simulink model "elevation_model"  (R2021b)
settings: Solver=VariableStepAuto  StartTime=0.0  StopTime=45  RelTol=1e-3
values from neighbouring files (symbols this model uses):
  ts3 = 10^-3    (= 0.001)    [loading_project.m]
libraries: simulink x3
settings Model: Creator=noait  LastModifiedBy=noait

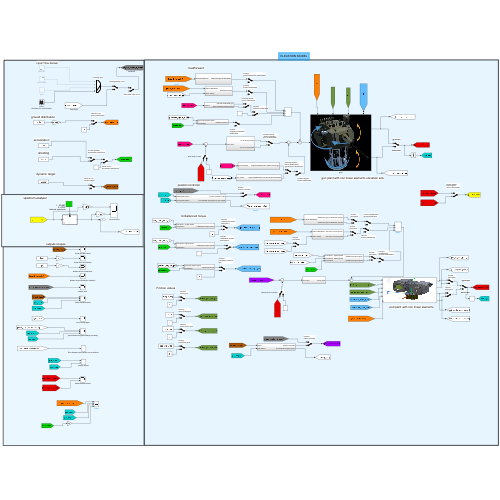
[thumbnail: Simulink's stored preview of the top-level diagram]
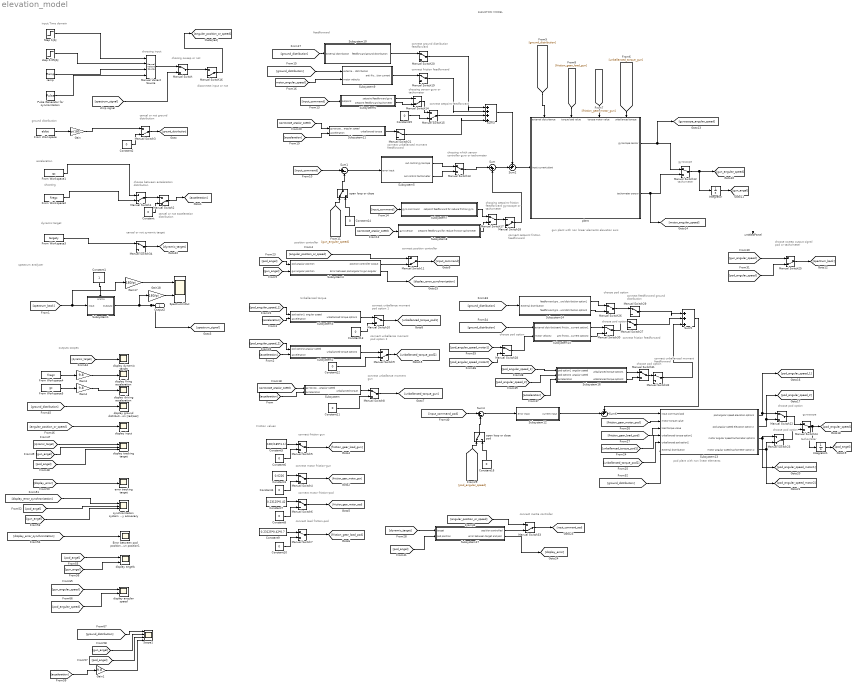
== system elevation_model ==
  note: ELEVATION MODEL
  note: outputs scopes
  note: connect
      | friction feedforward
  note: connect feedforward
      | ground distribution
  note: choose
      | pod option
  note: connect
      | unballance moment
      | pod option 2
  note: connect
      | inertia controller
  note: connect
      | motor friction-gun
  note: connect
      | friction gun
  note: choose sweep
      | output signal
      |  pod or tachometer
  note: connect
      | position controller
  note: connect setpoint
      | friction feedforward
  note: chossing setpoint
      | friction feedforward
      |  gyroscope or tachometer
  note: chossing which
      |  sensor controller
      | gyro or tachometer
  note: chossing sensor
      | gyro or tachometer
  note: connect
      | ground distribution feedforward
  note: disconnect input or not
  note: chosing sweep or not
  note: choosing input
  note: cancel or not
      | synamic target
  note: cancel or not
      | ground distribution
  note: cancel or not
      | acceleration distribution
  note: choose between
      | acceleration distribution
  note: pod plant with non linear elements
  note: dynamic target
  note: feedforward
  note: shooting
  note: position controller
  note: gun plant with non linear elements elevation axis
  note: tachometer
  note: gyroscope
  note: Unballanced torque
  note: Friction values
  note: acceleration
  note: ground distribution
  note: spectrum analyzer
  note: input:Time domain
  note: connect
      | friction feedforward
  note: connect
      | setpoint feedforward
  note: connect
      | unballanced moment
      | feedforward
  note: connect
      | motor friction-pod
  note: connect
      | load friction-pod
  note: connect
      | unballance moment
      | pod option 1
  note: connect
      | unballance moment
      | gun
  note: choose
      | pod option
  note: choose
      | pod option
  note: choose
      | pod option
  note: connect
      | unballanced
      | moment feedforward
  note: choose
      | pod option
  note: choose
      | pod option
  note: gyroscope
  note: tachometer
  " synchronization system stability accuaracy" : Scope  NumInputPorts=3
  Constant : Constant  Value=0  SampleTime=-1
  Constant1 : Constant  OutDataTypeStr=boolean
      settings: AttributesFormatString=1 - START\n0 -STOP\ninternal spectrum
      settings: OpenFcn=|
      | if get_param(gcbh,'value')-48 set_param(gcbh,'value','0','backgroundcolor','red');
      | else set_param(gcbh,'value','1','backgroundcolor','green');
      | end
  Constant{4,6,8,10..16} (10 alike) : Constant  Value=0  SampleTime=0
  Constant2 : Constant  Value=0  SampleTime=-1
  Constant3 : Constant  Value=0.0226  SampleTime=0
  Constant5 : Constant  Value=100/(185*1.1)  SampleTime=0
  Constant7 : Constant  Value=0.23125*0.42  SampleTime=0
  Constant9 : Constant  Value=0.23125*0.42*0.7  SampleTime=0
  Error between pod position to gun position1 : Scope
  From Workspace : FromWorkspace  VariableName=eldist  SampleTime=ts3/3  Interpolate=off  ZeroCross=off  OutputAfterFinalValue=Setting to zero
  From Workspace1 : FromWorkspace  VariableName=gz  SampleTime=ts3/3  Interpolate=off  ZeroCross=off  OutputAfterFinalValue=Setting to zero
  From Workspace2 : FromWorkspace  VariableName=firegz  SampleTime=ts3/9  Interpolate=off  ZeroCross=off  OutputAfterFinalValue=Setting to zero
  From Workspace3 : FromWorkspace  VariableName=targety  SampleTime=5*ts3  Interpolate=off  ZeroCross=off  OutputAfterFinalValue=Setting to zero
  From Workspace4 : FromWorkspace  VariableName=firegz  SampleTime=ts3/9  Interpolate=off  ZeroCross=off  OutputAfterFinalValue=Setting to zero
  From Workspace5 : FromWorkspace  VariableName=gz  SampleTime=ts3/3  Interpolate=off  ZeroCross=off  OutputAfterFinalValue=Setting to zero
  Gain : Gain  Gain=pi/180
  Gain1 : Gain  Gain=9.8
  Gain17 : Gain  Gain=180/pi
  Gain18 : Gain  Gain=180/pi
  Gain3 : Gain  Gain=9.8
  Gain4 : Gain  Gain=9.8
  Integrator : Integrator  ZeroCross=off
  Integrator1 : Integrator  ZeroCross=off
  Manual Variant Source : simulink/Signal Routing/Manual Variant Source  NumChoices=4  LabelModeActiveChoice=V_4
  Manual Switch{,4..8,10,12..13,17,19..22,24,26..32,34} (23 alike) : ManualSwitch
  Manual Switch{1..3,9,11,14..16,18,23,25,33} (12 alike) : ManualSwitch  CurrentSetting=0
  Pulse Generator for syncronization : DiscretePulseGenerator  PulseType=Time based  Period=5  PulseWidth=20
  Scope1 : Scope  NumInputPorts=4
  SpectrumInOut : Scope  NumInputPorts=2
  Step 1[A] : Step  SampleTime=0  ZeroCross=off
  Subsystem : Subsystem
  Subsystem1 : Subsystem  mask{GAIN=0.05%2*pi/180%0.5*pi/180, InitFreq=1, TargetTime=500, FreqAtTime=500}
      mask prompts: InitFreq "INITIAL FREQUENCY"; TargetTime "Target Time"; FreqAtTime "Frequency at Time"
  Subsystem10 : Subsystem
  Subsystem11 : Subsystem
  Subsystem12 : Subsystem
  Subsystem13 : Subsystem
      mask Display: image('C:\Users\noait\OneDrive\Desktop\צילום מסך 2024-04-08 195106.png'); % Use "Edit Image" on toolstrip to change.
  Subsystem14 : Subsystem
  Subsystem15 : Subsystem
  Subsystem16 : Subsystem
  Subsystem17 : Subsystem
  Subsystem2 : Subsystem
  Subsystem3 : Subsystem
  Subsystem4 : Subsystem
  Subsystem5 : Subsystem
  Subsystem6 : Subsystem
  Subsystem7 : Subsystem
  Subsystem8 : Subsystem
  Subsystem9 : Subsystem
  Sum : Sum  Inputs=|++
  Sum1 : Sum  Inputs=|+-
  Sum2 : Sum  Inputs=++|
  Sum3 : Sum  Inputs=|++++
  Sum4 : Sum  Inputs=|+-
  Sum5 : Sum  Inputs=|+++
  Sum6 : Sum  Inputs=++|
  display angels : Scope  NumInputPorts=2
  display angular speed : Scope  NumInputPorts=2
  display driving acceleration : Scope
  display dynamic target : Scope
  display firing acceleration : Scope
  display ground distribution [rad/sec] : Scope
  display input : Scope
  display tracking target : Scope  NumInputPorts=3
  error tracking target : Scope
  open loop or close : ManualSwitch
  open loop or close pod : ManualSwitch
  plant : Subsystem  Description=elevation-plant
      settings: PortSchema="{\"entries\":[{\"content\":{\"sides\":[{\"content\":{\"connectorIds\":[\"In1\"]},\"type\":\"ConnectorPlacement.EquallySpacedRectSide\",\"uuid\":\"e984d65b-c4b2-4f64-9138-3f858c9b51b0\"},{\"content\":{\"connectorIds\":[\"Out1\",\"Out2\"],\"side\":\"RIGHT\"},\"type\":\"ConnectorPlacement.EquallySpacedRectSide\",\"uuid\":\"67e0a38d-5f11-4d68-ba2b-c2f31a8ec962\"},{\"content\":{\"connectorIds\":[\"In2\",\"In3\",\"In4\",\"In5\"],\"side\":\"TOP\"},\"type\":\"ConnectorPlacement.EquallySpacedRectSide\",\"uuid\":\"636aa855-affb-4e96-b788-9501fa5a8af5\"}]},\"type\":\"ConnectorPlacement.EquallySpacedConnector\",\"uuid\":\"459d9826-6541-4e32-b3aa-984fb23680a1\"}],\"packageUris\":[\"http://schema.mathworks.com/mf0/Connector/R2020b\"],\"version\":\"1.0\"}"
      mask Display: image('C:\Users\noait\OneDrive\Desktop\צילום.png'); % Use "Edit Image" on toolstrip to change.
  ramp : simulink/Sources/Ramp  slope=1  start=0  InitialOutput=0
  step 0.05[A] : Step  After=0.05  SampleTime=0  ZeroCross=off
  untitledPanel : Subsystem  Tag=HiddenForWebPanel  IsWebBlockPanel=on
  Output2 : Outport
  wires:
  ramp/1 -> Manual Variant Source/3
  Step 1[A]/1 -> Manual Variant Source/1
  Pulse Generator for syncronization/1 -> Manual Variant Source/4
  step 0.05[A]/1 -> Manual Variant Source/2
  Manual Variant Source/1 -> Manual Switch/1
  Gain17/1 -> SpectrumInOut/1
  Constant1/1 -> Subsystem1/Enable
  Subsystem1/1(Output2) -> [spectrum_signal], Output2/1, Gain18/1
  [spectrum_back] -> Gain17/1, Subsystem1/1(Input)
  Gain18/1 -> SpectrumInOut/2
  [spectrum_signal] -> Manual Switch/2
  From Workspace/1 -> Gain/1
  Gain/1 -> Manual Switch3/1
  From Workspace1/1 -> Manual Switch1/1
  From Workspace2/1 -> Manual Switch1/2
  Manual Switch1/1 -> Manual Switch2/1
  Manual Switch2/1 -> [acceleration]
  Constant/1 -> Manual Switch2/2
  Manual Switch3/1 -> [ground_distribution]
  Constant2/1 -> Manual Switch3/2
  Constant3/1 -> Manual Switch4/1
  Constant4/1 -> Manual Switch4/2
  Manual Switch4/1 -> [friction_gear_motor_gun]
  Constant5/1 -> Manual Switch5/1
  Manual Switch5/1 -> [friction_gear_load_gun]
  Constant6/1 -> Manual Switch5/2
  Constant7/1 -> Manual Switch6/1
  Manual Switch6/1 -> [friction_gear_motor_pod]
  Constant8/1 -> Manual Switch6/2
  Manual Switch7/1 -> [friction_gear_load_pod]
  Constant10/1 -> Manual Switch7/2
  Constant9/1 -> Manual Switch7/1
  [acceleration] -> Subsystem/2(acceleration)
  Manual Switch8/1 -> [unballanced_torque_gun]
  Subsystem/1(unballanced torque) -> Manual Switch8/1
  Constant11/1 -> Manual Switch8/2
  Constant12/1 -> Manual Switch9/2
  [acceleration] -> Subsystem2/2(acceleration)
  Subsystem2/1(unballanced torque option2) -> Manual Switch9/1
  Constant13/1 -> Manual Switch10/2
  [acceleration] -> Subsystem3/2(acceleration)
  Subsystem3/1(unballanced torque option1) -> Manual Switch10/1
  Manual Switch10/1 -> [unballanced_torque_pod1]
  Manual Switch9/1 -> [unballanced_torque_pod2]
  Subsystem4/1(position controller output) -> Manual Switch11/2
  [angular_position_or_speed] -> Manual Switch11/1
  Manual Switch11/1 -> [input_command]
  [unballanced_torque_gun] -> plant/5(unballanced torque)
  [friction_gear_motor_gun] -> plant/4(torque motor value)
  [friction_gear_load_gun] -> plant/3(torque load value)
  plant/2(tachometer sensor) -> [motor_angular_speed], Manual Switch12/2
  plant/1(gyroscope sensor) -> [gyroscope_angular_speed], Manual Switch12/1
  Manual Switch12/1 -> Integrator/1, [gun_angular_speed]
  Integrator/1 -> [gun_angel]
  [gun_angel] -> Subsystem4/2(gun angular position)
  Subsystem5/1(out control gyroscope) -> Manual Switch13/1
  Subsystem5/2(out control tachometer) -> Manual Switch13/2
  Sum1/1 -> Subsystem5/1(error input)
  [input_command] -> Sum1/1
  open loop or close/1 -> Sum1/2
  [gun_angular_speed] -> open loop or close/1
  Constant14/1 -> open loop or close/2
  Subsystem6/1(setpoind feedforward gyro) -> Manual Switch14/1
  Subsystem6/2(setpoint feedforward tachometer) -> Manual Switch14/2
  Manual Switch14/1 -> Manual Switch15/1
  Constant15/1 -> Manual Switch15/2
  Manual Switch/1 -> Manual Switch16/1
  Manual Switch16/1 -> [angular_position_or_speed]
  Sum/1 -> Sum2/2
  Sum2/1 -> plant/1(input current plant)
  [gyroscope_angular_speed] -> Subsystem8/1(gyro sensor)
  Subsystem8/1(setpoint feedforward for reduce friction tachometer) -> Manual Switch17/2
  Subsystem7/1(setpoint feedforward for reduce friction gyro) -> Manual Switch17/1
  Manual Switch17/1 -> Manual Switch18/1
  Manual Switch13/1 -> Sum/1
  Manual Switch18/1 -> Sum/2
  [input_command] -> Subsystem6/1(setpoint)
  [input_command] -> Subsystem7/1(gyro command)
  [ground_distribution] -> Subsystem9/1(external distribution)
  Subsystem9/1(anti friction current) -> Manual Switch19/1
  Sum3/1 -> Sum2/1
  [motor_angular_speed] -> Subsystem9/2(motor velocity)
  [ground_distribution] -> Subsystem10/1(external distribution)
  Subsystem10/1(feedforward ground distribution) -> Manual Switch20/1
  Manual Switch20/1 -> Sum3/1
  Manual Switch19/1 -> Sum3/2
  Manual Switch15/1 -> Sum3/3
  [gyroscope_angular_speed] -> Subsystem/1(gyroscope angular speed)
  [gyroscope_angular_speed] -> Subsystem11/1(gyroscope angular speed)
  [acceleration] -> Subsystem11/2(acceleration)
  Subsystem11/1(unballanced torque) -> Manual Switch21/1
  Manual Switch21/1 -> Sum3/4
  Subsystem13/1(pod angular speed elevation option1) -> [pod_angular_speed_1], Manual Switch22/1
  Subsystem13/2(pod angular speed elevation option 2) -> [pod_angular_speed_2], Manual Switch22/2
  Subsystem13/3(motor angular speed tachometer option1) -> Manual Switch23/1, [pod_angular_speed_motor1]
  Subsystem13/4("motor angular speed tachometer option 2 ") -> [pod_angular_speed_motor2], Manual Switch23/2
  [pod_angular_speed_1] -> Subsystem3/1("pod option1  angular speed ")
  [pod_angular_speed_2] -> Subsystem2/1(pod option2 angular speed)
  Manual Switch22/1 -> Manual Switch24/1
  Manual Switch23/1 -> Manual Switch24/2
  Manual Switch24/1 -> Integrator1/1, [pod_angular_speed]
  [pod_angel] -> Subsystem4/1(pod angular position)
  [unballanced_torque_pod1] -> Subsystem13/4(unballanced torque option1)
  [unballanced_torque_pod2] -> Subsystem13/5(unballanced pod option2)
  [friction_gear_motor_pod] -> Subsystem13/2(motor torque value)
  [friction_gear_load_pod] -> Subsystem13/3(load torque value)
  Constant16/1 -> open loop or close pod/2
  [pod_angular_speed] -> open loop or close pod/1
  Sum4/1 -> Subsystem12/1(error input)
  open loop or close pod/1 -> Sum4/2
  Manual Switch25/1 -> [spectrum_back]
  [gun_angular_speed] -> Manual Switch25/1
  [pod_angular_speed] -> Manual Switch25/2
  [ground_distribution] -> Subsystem13/6(external distribution)
  Subsystem14/1(feedforward ground distribution option1) -> Manual Switch26/1
  [ground_distribution] -> Subsystem14/1(external distribution)
  Sum6/1 -> Subsystem13/1(input command pod)
  Subsystem12/1(current input) -> Sum6/2
  Sum5/1 -> Sum6/1
  [ground_distribution] -> Subsystem15/1(external distribution)
  Manual Switch27/1 -> Sum5/2
  [pod_angular_speed_motor1] -> Manual Switch28/1
  Manual Switch28/1 -> Subsystem15/2(motor velocity)
  [pod_angular_speed_motor2] -> Manual Switch28/2
  Subsystem14/2(feedforward ground distribution option2) -> Manual Switch26/2
  Manual Switch26/1 -> Manual Switch29/1
  Manual Switch29/1 -> Sum5/1
  Subsystem15/1(anti friction current option1) -> Manual Switch30/1
  Subsystem15/2(anti friction current option2) -> Manual Switch30/2
  Manual Switch30/1 -> Manual Switch27/1
  [acceleration] -> Subsystem16/3(acceleration)
  [pod_angular_speed_1] -> Subsystem16/1("pod option1  angular speed ")
  [pod_angular_speed_2] -> Subsystem16/2("pod option2  angular speed ")
  Subsystem16/1(unballanced torque option1) -> Manual Switch31/1
  Subsystem16/2(unballanced torque option2) -> Manual Switch31/2
  Manual Switch31/1 -> Manual Switch32/1
  Manual Switch32/1 -> Sum5/3
  Subsystem4/2(Error between pod angular to gun angular) -> [display_error_synchronization]
  From Workspace3/1 -> Manual Switch34/1
  [pod_angel] -> Subsystem17/2(pod position)
  Subsystem17/1(position controlled) -> Manual Switch33/2
  [angular_position_or_speed] -> Manual Switch33/1
  Manual Switch33/1 -> [input_command_pod]
  [input_command_pod] -> Sum4/1
  [dynamic_target] -> Subsystem17/1(target)
  [ground_distribution] -> plant/2(external disturbance)
  Integrator1/1 -> [pod_angel]
  Manual Switch34/1 -> [dynamic_target]
  [dynamic_target] -> display dynamic target/1
  Gain3/1 -> display firing acceleration/1
  From Workspace4/1 -> Gain3/1
  From Workspace5/1 -> Gain4/1
  Gain4/1 -> display driving acceleration/1
  [ground_distribution] -> display ground distribution [rad/sec]/1
  [angular_position_or_speed] -> display input/1
  [gun_angel] -> display tracking target/2
  [dynamic_target] -> display tracking target/1
  [pod_angel] -> display tracking target/3
  Subsystem17/2(error between target and pod) -> [display_error]
  [display_error] -> error tracking target/1
  [display_error_synchronization] -> " synchronization system stability accuaracy"/1
  [pod_angel] -> " synchronization system stability accuaracy"/2
  [gun_angel] -> " synchronization system stability accuaracy"/3
  [display_error_synchronization] -> Error between pod position to gun position1/1
  [pod_angel] -> display angels/1
  [gun_angel] -> display angels/2
  [gun_angular_speed] -> display angular speed/1
  [pod_angular_speed] -> display angular speed/2
  [ground_distribution] -> Scope1/1
  [gun_angel] -> Scope1/2
  [pod_angel] -> Scope1/3
  [acceleration] -> Gain1/1
  Gain1/1 -> Scope1/4

== system elevation_model/Subsystem ==
  gyroscope angular speed : Inport
  acceleration : Inport  Port=2
  Constant : Constant  SampleTime=-1
  Cos1 : Trigonometry  Operator=cos
  Gain3 : Gain  Gain=100/185
  Integrator : Integrator  ZeroCross=off
  Product : Product
  Sum : Sum  Inputs=|++
  unballanced torque : Outport
  wires:
  Gain3/1 -> unballanced torque/1
  Product/1 -> Gain3/1
  Cos1/1 -> Product/1
  acceleration/1 -> Sum/1
  Sum/1 -> Product/2
  Constant/1 -> Sum/2
  Integrator/1 -> Cos1/1
  gyroscope angular speed/1 -> Integrator/1

== system elevation_model/Subsystem1 ==
  Input : Inport
  Enable : EnablePort  StatesWhenEnabling=reset
  Chirp Signal1 : simulink/Sources/Chirp Signal  f1=1  T=160  f2=160
  Mux2 : Mux  Inputs=2
  Scope2 : Scope
  TSABAD_out_log : Scope
  gain 3 : Gain  Gain=GAIN  SaturateOnIntegerOverflow=on  SampleTime=ts3  OutDataTypeStr=Inherit: Same as input  ParamDataTypeStr=Inherit: Same as input
  Output2 : Outport
  wires:
  gain 3/1 -> Output2/1, Mux2/1
  Input/1 -> Mux2/2
  Mux2/1 -> TSABAD_out_log/1
  Chirp Signal1/1 -> gain 3/1, Scope2/1

== system elevation_model/Subsystem10 ==
  external distribution : Inport
  Gain3 : Gain  Gain=-1
  Transfer Fcn1 : TransferFcn  Numerator="[0.003753 0.1609 350.7  0]"  Denominator=[0.001592 1.064 178.8 8.72*10^4]
  feedforward ground distribution : Outport
  wires:
  Gain3/1 -> feedforward ground distribution/1
  Transfer Fcn1/1 -> Gain3/1
  external distribution/1 -> Transfer Fcn1/1

== system elevation_model/Subsystem11 ==
  gyroscope angular speed : Inport
  acceleration : Inport  Port=2
  Constant : Constant  SampleTime=-1
  Cos1 : Trigonometry  Operator=cos
  Gain : Gain  Gain=1/8.282809728
  Gain1 : Gain  Gain=sqrt(3)/0.39
  Gain3 : Gain  Gain=100/185
  Integrator : Integrator  ZeroCross=off
  Product : Product
  Sum : Sum  Inputs=|++
  unballanced torque : Outport
  wires:
  Product/1 -> Gain3/1
  Cos1/1 -> Product/1
  acceleration/1 -> Sum/1
  Sum/1 -> Product/2
  Constant/1 -> Sum/2
  Integrator/1 -> Cos1/1
  gyroscope angular speed/1 -> Integrator/1
  Gain1/1 -> Gain/1
  Gain3/1 -> Gain1/1
  Gain/1 -> unballanced torque/1

== system elevation_model/Subsystem12 ==
  error input : Inport
  Gain : Gain  Gain=136
  Gain4 : Gain  Gain=2*pi*1
  Gain5 : Gain
  Integrator1 : Integrator
  Sum2 : Sum  Inputs=|++
  current input : Outport
  wires:
  error input/1 -> Gain/1
  Integrator1/1 -> Sum2/1
  Gain4/1 -> Integrator1/1
  Gain/1 -> Gain4/1, Gain5/1
  Gain5/1 -> Sum2/2
  Sum2/1 -> current input/1

== system elevation_model/Subsystem13 ==
  input command pod : Inport
  motor torque value : Inport  Port=2
  load torque value : Inport  Port=3
  unballanced torque option1 : Inport  Port=4
  unballanced pod option2 : Inport  Port=5
  external distribution : Inport  Port=6
  " plant pod elevation  option 1" : Subsystem
  " plant pod elevation option 2" : Subsystem
  Saturation4 : Saturate  UpperLimit=11.933*sqrt(10)/1.59  LowerLimit=-11.933*sqrt(10)/1.59  ZeroCross=off
  Saturation6 : Saturate  UpperLimit=11.933*sqrt(10)*0.5/(1.59*0.52)  LowerLimit=-11.933*sqrt(10)*0.5/(1.59*0.52)  ZeroCross=off
  pod angular speed elevation option1 : Outport
  pod angular speed elevation option 2 : Outport  Port=2
  motor angular speed tachometer option1 : Outport  Port=3
  "motor angular speed tachometer option 2 " : Outport  Port=4
  wires:
  Saturation4/1 -> " plant pod elevation option 2"/1(current input)
  Saturation6/1 -> " plant pod elevation  option 1"/1(current input)
  input command pod/1 -> Saturation4/1, Saturation6/1
  " plant pod elevation  option 1"/1(pod angular speed elevation) -> pod angular speed elevation option1/1
  " plant pod elevation option 2"/1(pod angular speed elevation) -> pod angular speed elevation option 2/1
  " plant pod elevation  option 1"/2("motor angular speed tachometer ") -> motor angular speed tachometer option1/1
  " plant pod elevation option 2"/2("motor angular speed tachometer ") -> "motor angular speed tachometer option 2 "/1
  motor torque value/1 -> " plant pod elevation option 2"/3(motor torque value), " plant pod elevation  option 1"/3(motor torque value pod)
  load torque value/1 -> " plant pod elevation  option 1"/4(torque load value pod), " plant pod elevation option 2"/4(load torque vaue)
  unballanced torque option1/1 -> " plant pod elevation  option 1"/2(unballanced torque option1)
  unballanced pod option2/1 -> " plant pod elevation option 2"/2(unballanced pod option2)
  external distribution/1 -> " plant pod elevation option 2"/5(external distribution), " plant pod elevation  option 1"/5(external distribution)

== system elevation_model/Subsystem14 ==
  external distribution : Inport
  Gain21 : Gain  Gain=1/1.057
  Gain22 : Gain  Gain=0.015
  Gain23 : Gain  Gain=sqrt(10)/1.59
  Gain3 : Gain  Gain=-1
  Gain41 : Gain  Gain=sqrt(10)*0.5/(1.59*0.52)
  Transfer Fcn2 : TransferFcn  Numerator=[1 0]  Denominator=[1/(2*pi*100) 1]
  feedforward ground distribution option1 : Outport
  feedforward ground distribution option2 : Outport  Port=2
  wires:
  Gain22/1 -> Gain3/1
  Gain21/1 -> Gain22/1
  external distribution/1 -> Transfer Fcn2/1
  Transfer Fcn2/1 -> Gain21/1
  Gain41/1 -> feedforward ground distribution option1/1
  Gain3/1 -> Gain23/1, Gain41/1
  Gain23/1 -> feedforward ground distribution option2/1

== system elevation_model/Subsystem15 ==
  external distribution : Inport
  motor velocity : Inport  Port=2
  Gain2 : Gain  Gain=0.23125*0.42*0.7
  Gain21 : Gain  Gain=1/1.057
  Gain23 : Gain  Gain=sqrt(10)/1.59
  Gain3 : Gain  Gain=-1
  Gain4 : Gain  Gain=100
  Gain41 : Gain  Gain=sqrt(10)*0.5/(1.59*0.52)
  Gain6 : Gain  Gain=100
  Gain7 : Gain  Gain=0.23125*0.42
  Sum : Sum  Inputs=|++
  Tanh : Trigonometry  Operator=tanh
  Tanh1 : Trigonometry  Operator=tanh
  anti friction current option1 : Outport
  anti friction current option2 : Outport  Port=2
  wires:
  external distribution/1 -> Gain3/1
  Gain3/1 -> Gain4/1
  Gain4/1 -> Tanh/1
  Tanh/1 -> Gain2/1
  Tanh1/1 -> Gain7/1
  Gain6/1 -> Tanh1/1
  motor velocity/1 -> Gain6/1
  Gain7/1 -> Sum/2
  Gain2/1 -> Sum/1
  Sum/1 -> Gain21/1
  Gain41/1 -> anti friction current option1/1
  Gain21/1 -> Gain23/1, Gain41/1
  Gain23/1 -> anti friction current option2/1

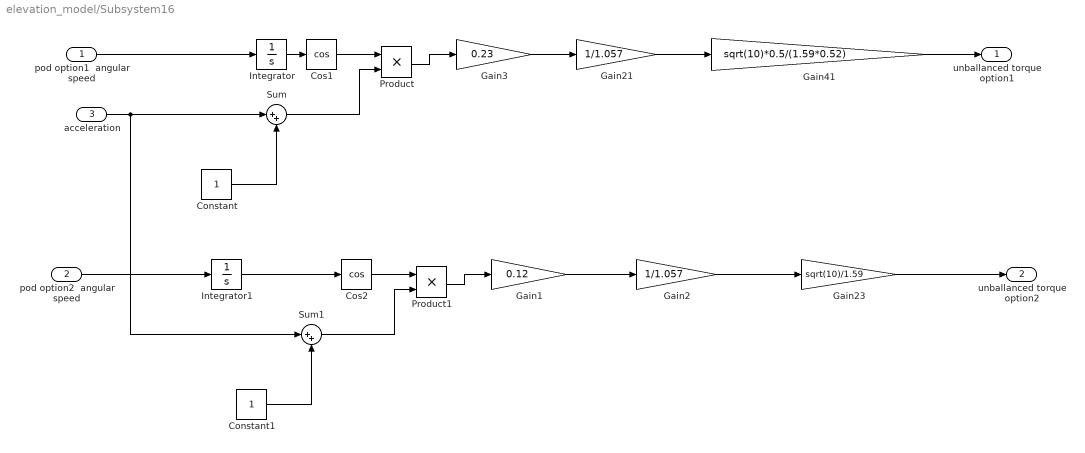
== system elevation_model/Subsystem16 ==
  "pod option1  angular speed " : Inport
  "pod option2  angular speed " : Inport  Port=2
  acceleration : Inport  Port=3
  Constant : Constant  SampleTime=-1
  Constant1 : Constant  SampleTime=-1
  Cos1 : Trigonometry  Operator=cos
  Cos2 : Trigonometry  Operator=cos
  Gain1 : Gain  Gain=0.12
  Gain2 : Gain  Gain=1/1.057
  Gain21 : Gain  Gain=1/1.057
  Gain23 : Gain  Gain=sqrt(10)/1.59
  Gain3 : Gain  Gain=0.23
  Gain41 : Gain  Gain=sqrt(10)*0.5/(1.59*0.52)
  Integrator : Integrator  ZeroCross=off
  Integrator1 : Integrator  ZeroCross=off
  Product : Product
  Product1 : Product
  Sum : Sum  Inputs=|++
  Sum1 : Sum  Inputs=|++
  unballanced torque option1 : Outport
  unballanced torque option2 : Outport  Port=2
  wires:
  Integrator/1 -> Cos1/1
  acceleration/1 -> Sum1/1, Sum/1
  "pod option1  angular speed "/1 -> Integrator/1
  Sum/1 -> Product/2
  Product/1 -> Gain3/1
  Cos1/1 -> Product/1
  Constant/1 -> Sum/2
  Gain3/1 -> Gain21/1
  Gain21/1 -> Gain41/1
  Gain41/1 -> unballanced torque option1/1
  Integrator1/1 -> Cos2/1
  Sum1/1 -> Product1/2
  Constant1/1 -> Sum1/2
  Gain1/1 -> Gain2/1
  Product1/1 -> Gain1/1
  Cos2/1 -> Product1/1
  "pod option2  angular speed "/1 -> Integrator1/1
  Gain2/1 -> Gain23/1
  Gain23/1 -> unballanced torque option2/1

== system elevation_model/Subsystem17 ==
  target : Inport
  pod position : Inport  Port=2
  Gain : Gain  Gain=30
  Gain1 : Gain  Gain=30
  Gain2 : Gain  Gain=-0.04
  Integrator1 : Integrator
  Sum : Sum  Inputs=|+-
  Sum1 : Sum  Inputs=|+++
  Transfer Fcn : TransferFcn  Numerator=[1 0]  Denominator=[1/(2*pi*100) 1]
  position controlled : Outport
  error between target and pod : Outport  Port=2
  wires:
  target/1 -> Sum/1
  pod position/1 -> Gain2/1, Sum/2
  Sum/1 -> error between target and pod/1, Gain1/1, Gain/1
  Integrator1/1 -> Sum1/1
  Gain1/1 -> Sum1/2
  Gain2/1 -> Transfer Fcn/1
  Transfer Fcn/1 -> Sum1/3
  Gain/1 -> Integrator1/1
  Sum1/1 -> position controlled/1

== system elevation_model/Subsystem2 ==
  pod option2 angular speed : Inport
  acceleration : Inport  Port=2
  Constant : Constant  SampleTime=-1
  Cos1 : Trigonometry  Operator=cos
  Gain3 : Gain  Gain=0.12
  Integrator : Integrator  ZeroCross=off
  Product : Product
  Sum : Sum  Inputs=|++
  unballanced torque option2 : Outport
  wires:
  Gain3/1 -> unballanced torque option2/1
  Product/1 -> Gain3/1
  Cos1/1 -> Product/1
  acceleration/1 -> Sum/1
  Sum/1 -> Product/2
  Constant/1 -> Sum/2
  pod option2 angular speed/1 -> Integrator/1
  Integrator/1 -> Cos1/1

== system elevation_model/Subsystem3 ==
  "pod option1  angular speed " : Inport
  acceleration : Inport  Port=2
  Constant : Constant  SampleTime=-1
  Cos1 : Trigonometry  Operator=cos
  Gain3 : Gain  Gain=0.23
  Integrator : Integrator  ZeroCross=off
  Product : Product
  Sum : Sum  Inputs=|++
  unballanced torque option1 : Outport
  wires:
  Gain3/1 -> unballanced torque option1/1
  Product/1 -> Gain3/1
  Cos1/1 -> Product/1
  acceleration/1 -> Sum/1
  Sum/1 -> Product/2
  Constant/1 -> Sum/2
  Integrator/1 -> Cos1/1
  "pod option1  angular speed "/1 -> Integrator/1

== system elevation_model/Subsystem4 ==
  pod angular position : Inport
  gun angular position : Inport  Port=2
  Gain : Gain  Gain=15.4
  Gain1 : Gain  Gain=2*pi*1
  Integrator : Integrator  ZeroCross=off
  Sum : Sum  Inputs=|+-
  Sum1 : Sum  Inputs=|++
  position controller output : Outport
  Error between pod angular to gun angular : Outport  Port=2
  wires:
  pod angular position/1 -> Sum/1
  gun angular position/1 -> Sum/2
  Sum/1 -> Error between pod angular to gun angular/1, Gain/1
  Sum1/1 -> position controller output/1
  Gain/1 -> Sum1/2, Gain1/1
  Gain1/1 -> Integrator/1
  Integrator/1 -> Sum1/1

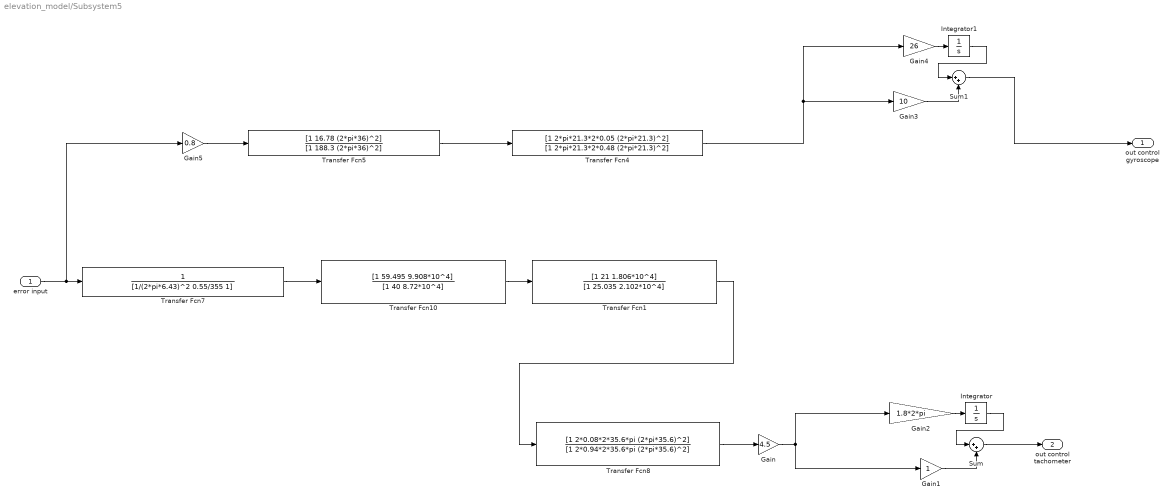
== system elevation_model/Subsystem5 ==
  error input : Inport
  Gain : Gain  Gain=4.5
  Gain1 : Gain
  Gain2 : Gain  Gain=1.8*2*pi
  Gain3 : Gain  Gain=10
  Gain4 : Gain  Gain=26
  Gain5 : Gain  Gain=0.8
  Integrator : Integrator
  Integrator1 : Integrator
  Sum : Sum  Inputs=|++
  Sum1 : Sum  Inputs=|++
  Transfer Fcn1 : TransferFcn  Numerator=[1 21 1.806*10^4]  Denominator=[1 25.035 2.102*10^4]
  Transfer Fcn10 : TransferFcn  Numerator=[1 59.495 9.908*10^4]  Denominator=[1 40 8.72*10^4]
  Transfer Fcn4 : TransferFcn  Numerator=[1 2*pi*21.3*2*0.05 (2*pi*21.3)^2]  Denominator=[1 2*pi*21.3*2*0.48 (2*pi*21.3)^2]
  Transfer Fcn5 : TransferFcn  Numerator=[1 16.78 (2*pi*36)^2]  Denominator=[1 188.3 (2*pi*36)^2]
  Transfer Fcn7 : TransferFcn  Denominator=[1/(2*pi*6.43)^2 0.55/355 1]
  Transfer Fcn8 : TransferFcn  Numerator=[1 2*0.08*2*35.6*pi (2*pi*35.6)^2]  Denominator=[1 2*0.94*2*35.6*pi (2*pi*35.6)^2]
  out control gyroscope : Outport
  out control tachometer : Outport  Port=2
  wires:
  Gain1/1 -> Sum/2
  Transfer Fcn10/1 -> Transfer Fcn1/1
  Transfer Fcn1/1 -> Transfer Fcn8/1
  Transfer Fcn8/1 -> Gain/1
  Gain2/1 -> Integrator/1
  Integrator/1 -> Sum/1
  Gain/1 -> Gain1/1, Gain2/1
  Sum/1 -> out control tachometer/1
  Transfer Fcn5/1 -> Transfer Fcn4/1
  Gain3/1 -> Sum1/2
  Integrator1/1 -> Sum1/1
  Gain4/1 -> Integrator1/1
  Transfer Fcn4/1 -> Gain3/1, Gain4/1
  Sum1/1 -> out control gyroscope/1
  Gain5/1 -> Transfer Fcn5/1
  error input/1 -> Transfer Fcn7/1, Gain5/1
  Transfer Fcn7/1 -> Transfer Fcn10/1

== system elevation_model/Subsystem6 ==
  setpoint : Inport
  setpoint feedforward gyro : TransferFcn  Numerator=[0.0006863 0.1022 118.6 1.043*10^4 5.355*10^6 1.9*10^8 6.014*10^10 0]  Denominator=[5.066*10^-6 0.008302 4.984 1642 4.448*10^5 7.498*10^7 4.289*10^9 5.4505*10^11]
  setpoint feedforward tacho : TransferFcn  Numerator=[1 148.9 1.729*10^5 1.52*10^7 7.802*10^9 2.769*10^11 8.762*10^13 0]  Denominator=[0.424 295 6.504*10^4 3.101*10^7 1.76*10^9 5.413*10^11 3.742*10^12 7.875*10^14]
  setpoind feedforward gyro : Outport
  setpoint feedforward tachometer : Outport  Port=2
  wires:
  setpoint/1 -> setpoint feedforward tacho/1, setpoint feedforward gyro/1
  setpoint feedforward gyro/1 -> setpoind feedforward gyro/1
  setpoint feedforward tacho/1 -> setpoint feedforward tachometer/1

== system elevation_model/Subsystem7 ==
  gyro command : Inport
  Gain : Gain  Gain=100
  Gain1 : Gain  Gain=100/(185*1.1)
  Tanh : Trigonometry  Operator=tanh
  Transfer Fcn : TransferFcn  Numerator=[0.006824 0.8287 1005 6.059*10^4 3.016*10^7]  Denominator=[0.001592 2.09 865 2.025*10^5 5.626*10^7]
  setpoint feedforward for reduce friction gyro : Outport
  wires:
  gyro command/1 -> Gain/1
  Gain/1 -> Tanh/1
  Tanh/1 -> Gain1/1
  Gain1/1 -> Transfer Fcn/1
  Transfer Fcn/1 -> setpoint feedforward for reduce friction gyro/1

== system elevation_model/Subsystem8 ==
  gyro sensor : Inport
  Gain : Gain  Gain=100
  Gain1 : Gain  Gain=100/(185*1.1)
  Tanh : Trigonometry  Operator=tanh
  Transfer Fcn : TransferFcn  Numerator=[2.932 1924 4.91*10^4 1.818*10^7]  Denominator=[1 27.24 2.26*10^4 9.157*10^4 3.39*10^7]
  setpoint feedforward for reduce friction tachometer : Outport
  wires:
  gyro sensor/1 -> Gain/1
  Gain/1 -> Tanh/1
  Tanh/1 -> Gain1/1
  Gain1/1 -> Transfer Fcn/1
  Transfer Fcn/1 -> setpoint feedforward for reduce friction tachometer/1

== system elevation_model/Subsystem9 ==
  external distribution : Inport
  motor velocity : Inport  Port=2
  Gain : Gain  Gain=1/8.282809728
  Gain1 : Gain  Gain=sqrt(3)/0.39
  Gain2 : Gain  Gain=100/(185*1.1)
  Gain3 : Gain  Gain=-1
  Gain4 : Gain  Gain=100
  Gain6 : Gain  Gain=100
  Gain7 : Gain  Gain=0.0226
  Sum : Sum  Inputs=|++
  Tanh : Trigonometry  Operator=tanh
  Tanh1 : Trigonometry  Operator=tanh
  anti friction current : Outport
  wires:
  Gain1/1 -> Gain/1
  Gain/1 -> anti friction current/1
  external distribution/1 -> Gain3/1
  Gain3/1 -> Gain4/1
  Gain4/1 -> Tanh/1
  Tanh/1 -> Gain2/1
  Gain2/1 -> Sum/1
  Sum/1 -> Gain1/1
  Tanh1/1 -> Gain7/1
  Gain6/1 -> Tanh1/1
  motor velocity/1 -> Gain6/1
  Gain7/1 -> Sum/2

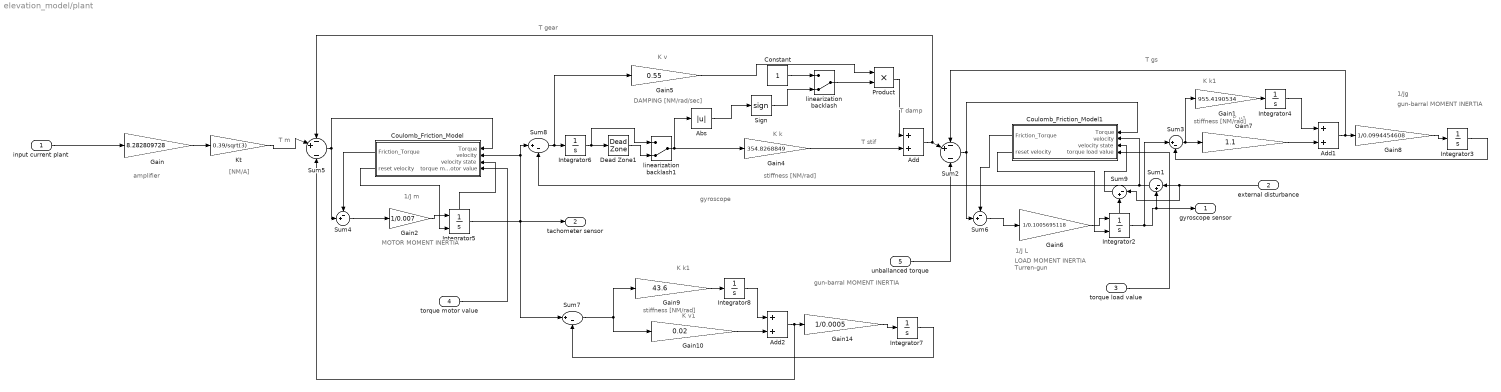
== system elevation_model/plant ==
  note: T gs
  note: [NM/A]
  note: K v
  note: amplifier
  note: DAMPING
      | [NM/rad/sec]
  note: K k1
  note: T damp
  note: K v1
  note: stiffness
      | [NM/rad]
  note: 1/J m
  note: MOTOR
      | MOMENT INERTIA
  note: T m
  note: 1/J L
  note: T stif
  note: K k
  note: T gear
  note: LOAD
      | MOMENT INERTIA
      | Turren-gun
  note: stiffness
      | [NM/rad]
  note: gyroscope
  note: gun-barral
      | MOMENT INERTIA
  note: 1/Jg
  note: K v1
  note: K k1
  note: stiffness
      | [NM/rad]
  note: gun-barral
      | MOMENT INERTIA
  input current plant : Inport
  external disturbance : Inport  Port=2
  torque load value : Inport  Port=3
  torque motor value : Inport  Port=4
  unballanced torque : Inport  Port=5
  Abs : Abs
  Add : Sum
  Add1 : Sum
  Add2 : Sum
  Constant : Constant
  Coulomb_Friction_Model : Subsystem
  Coulomb_Friction_Model1 : Subsystem
  Dead Zone1 : DeadZone  LowerValue=-0.07*10^-3  UpperValue=0.07*10^-3  ZeroCross=off
  Gain : Gain  Gain=8.282809728
  Gain1 : Gain  Gain=955.4190534
  Gain10 : Gain  Gain=0.02
  Gain14 : Gain  Gain=1/0.0005
  Gain2 : Gain  Gain=1/0.007
  Gain4 : Gain  Gain=354.8268849
  Gain5 : Gain  Gain=0.55
  Gain6 : Gain  Gain=1/0.1005695118
  Gain7 : Gain  Gain=1.1
  Gain8 : Gain  Gain=1/0.0994454608
  Gain9 : Gain  Gain=43.6
  Integrator2 : Integrator  ExternalReset=rising  ShowStatePort=on  ZeroCross=off
  Integrator{3..4,6..8} (5 alike) : Integrator
  Integrator5 : Integrator  ExternalReset=rising  ShowStatePort=on  ZeroCross=off
  Kt : Gain  Gain=0.39/sqrt(3)
  Product : Product
  Sign : Signum
  Sum1 : Sum  Inputs=|-+
  Sum2 : Sum  Inputs=-+|-
  Sum3 : Sum  Inputs=|+-
  Sum4 : Sum  Inputs=-+|
  Sum5 : Sum  Inputs=-+|-
  Sum6 : Sum  Inputs=-+|
  Sum7 : Sum  Inputs=|+-
  Sum8 : Sum  Inputs=|+-
  Sum9 : Sum  Inputs=|-+
  linearization backlash : ManualSwitch  CurrentSetting=0
  linearization backlash1 : ManualSwitch  CurrentSetting=0
  gyroscope sensor : Outport
  tachometer sensor : Outport  Port=2
  wires:
  Constant/1 -> linearization backlash/1
  Gain/1 -> Kt/1
  Add/1 -> Sum5/1, Sum2/2
  Integrator4/1 -> Add1/1
  Kt/1 -> Sum5/2
  Gain6/1 -> Integrator2/1
  Gain5/1 -> Product/1
  Gain4/1 -> Add/2
  Sum3/1 -> Gain7/1, Gain1/1
  Sum8/1 -> Gain5/1, Integrator6/1
  Gain2/1 -> Integrator5/1
  Product/1 -> Add/1
  Integrator6/1 -> linearization backlash1/1, Dead Zone1/1
  Abs/1 -> Sign/1
  Gain7/1 -> Add1/2
  linearization backlash/1 -> Product/2
  Integrator3/1 -> Sum3/2
  Sign/1 -> linearization backlash/2
  Gain1/1 -> Integrator4/1
  Sum4/1 -> Gain2/1
  Sum5/1 -> Coulomb_Friction_Model/1(Torque), Sum4/2
  Sum6/1 -> Gain6/1
  Gain8/1 -> Integrator3/1
  Add1/1 -> Gain8/1, Sum2/1
  Integrator2/1 -> Sum1/2, gyroscope sensor/1, Sum3/1
  input current plant/1 -> Gain/1
  Sum2/1 -> Sum6/2, Coulomb_Friction_Model1/1(Torque)
  Coulomb_Friction_Model/1(Friction_Torque) -> Sum4/1
  Integrator5/State -> Coulomb_Friction_Model/3(velocity state)
  Coulomb_Friction_Model/2(reset velocity) -> Integrator5/2
  Integrator8/1 -> Add2/1
  Gain9/1 -> Integrator8/1
  Gain10/1 -> Add2/2
  Gain14/1 -> Integrator7/1
  Add2/1 -> Sum5/3, Gain14/1
  Sum7/1 -> Gain10/1, Gain9/1
  Integrator7/1 -> Sum7/2
  linearization backlash1/1 -> Abs/1, Gain4/1
  Dead Zone1/1 -> linearization backlash1/2
  Coulomb_Friction_Model1/1(Friction_Torque) -> Sum6/1
  Coulomb_Friction_Model1/2(reset velocity) -> Integrator2/2
  Sum1/1 -> Coulomb_Friction_Model1/2(velocity), Sum8/2
  Integrator2/State -> Sum9/2
  Sum9/1 -> Coulomb_Friction_Model1/3(velocity state)
  Integrator5/1 -> tachometer sensor/1, Sum7/1, Coulomb_Friction_Model/2(velocity), Sum8/1
  external disturbance/1 -> Sum9/1, Sum1/1
  unballanced torque/1 -> Sum2/3
  torque motor value/1 -> Coulomb_Friction_Model/4(torque motor value)
  torque load value/1 -> Coulomb_Friction_Model1/4(torque load value)

== system elevation_model/untitledPanel ==
  Callback Button1 : CallbackButton  Tag=HiddenForWebPanel  PanelInfo="{\"panelId\":\"panelId-3d7ee8a4-1926-4a42-ae9e-9d07c4a1cb87\",\"type\":\"panelChild\",\"version\":\"2019b\",\"zIndex\":1500002}"
  panelInfo : PanelWebBlock  Tag=HiddenForWebPanel  PanelInfo="{\"compacted\":false,\"height\":84,\"isActiveTab\":true,\"left\":1069,\"name\":\"Panel\",\"panelId\":\"panelId-3d7ee8a4-1926-4a42-ae9e-9d07c4a1cb87\",\"tabIndex\":0,\"tabbedSetId\":\"tabbedSet8564127506\",\"top\":912,\"type\":\"panel\",\"version\":\"2019b\",\"visible\":true,\"width\":178,\"zIndex\":1500002}"

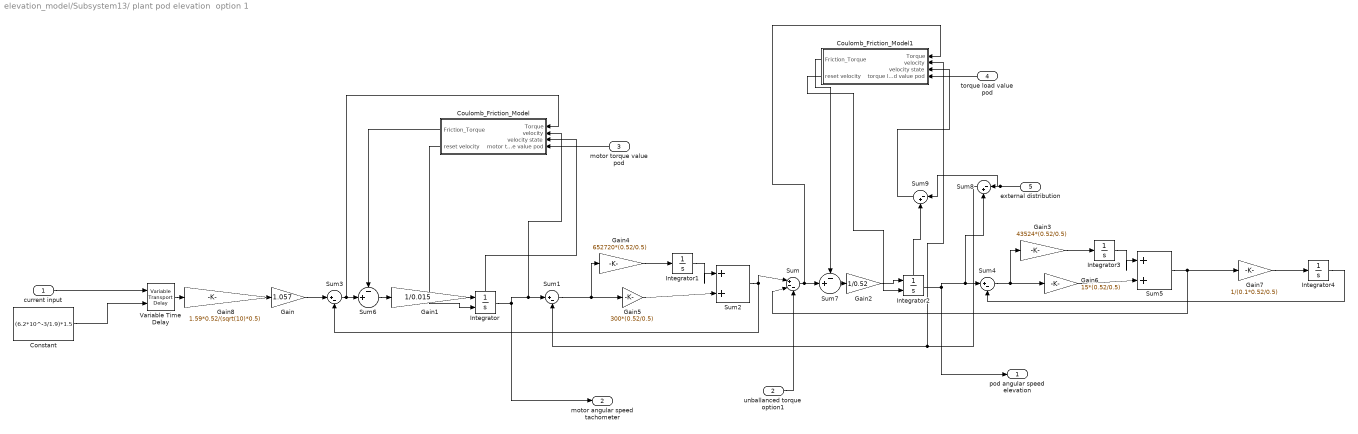
== system elevation_model/Subsystem13/ plant pod elevation  option 1 ==
  current input : Inport
  unballanced torque option1 : Inport  Port=2
  motor torque value pod : Inport  Port=3
  torque load value pod : Inport  Port=4
  external distribution : Inport  Port=5
  Constant : Constant  Value=(6.2*10^-3/1.9)*1.5  SampleTime=-1
  Coulomb_Friction_Model : Subsystem
  Coulomb_Friction_Model1 : Subsystem
  Gain : Gain  Gain=1.057
  Gain1 : Gain  Gain=1/0.015
  Gain2 : Gain  Gain=1/0.52
  Gain3 : Gain  Gain=43524*(0.52/0.5)
  Gain4 : Gain  Gain=652720*(0.52/0.5)
  Gain5 : Gain  Gain=300*(0.52/0.5)
  Gain6 : Gain  Gain=15*(0.52/0.5)
  Gain7 : Gain  Gain=1/(0.1*0.52/0.5)
  Gain8 : Gain  Gain=1.59*0.52/(sqrt(10)*0.5)
  Integrator : Integrator  ExternalReset=rising  ShowStatePort=on  ZeroCross=off
  Integrator1 : Integrator
  Integrator2 : Integrator  ExternalReset=rising  ShowStatePort=on  ZeroCross=off
  Integrator3 : Integrator
  Integrator4 : Integrator
  Sum : Sum  Inputs=|+--
  Sum1 : Sum  Inputs=|+-
  Sum2 : Sum  Inputs=|++
  Sum3 : Sum  Inputs=|+-
  Sum4 : Sum  Inputs=|+-
  Sum5 : Sum  Inputs=|++
  Sum6 : Sum  Inputs=-+|
  Sum7 : Sum  Inputs=-+|
  Sum8 : Sum  Inputs=|-+
  Sum9 : Sum  Inputs=|-+
  Variable Time Delay : VariableTransportDelay  MaximumDelay=10  TransDelayFeedthrough=on
  pod angular speed elevation : Outport
  "motor angular speed tachometer " : Outport  Port=2
  wires:
  Integrator3/1 -> Sum5/1
  Gain7/1 -> Integrator4/1
  Gain8/1 -> Gain/1
  Sum5/1 -> Gain7/1, Sum/2
  Gain6/1 -> Sum5/2
  Gain5/1 -> Sum2/2
  Integrator4/1 -> Sum4/2
  Gain/1 -> Sum3/1
  Sum1/1 -> Gain5/1, Gain4/1
  Sum4/1 -> Gain6/1, Gain3/1
  Integrator1/1 -> Sum2/1
  current input/1 -> Variable Time Delay/1
  Variable Time Delay/1 -> Gain8/1
  Constant/1 -> Variable Time Delay/2
  Sum2/1 -> Sum/1, Sum3/2
  Gain2/1 -> Integrator2/1
  Gain4/1 -> Integrator1/1
  Gain3/1 -> Integrator3/1
  Gain1/1 -> Integrator/1
  Integrator/1 -> Coulomb_Friction_Model/2(velocity), Sum1/1, "motor angular speed tachometer "/1
  Coulomb_Friction_Model/2(reset velocity) -> Integrator/2
  Sum3/1 -> Coulomb_Friction_Model/1(Torque), Sum6/2
  Integrator/State -> Coulomb_Friction_Model/3(velocity state)
  Coulomb_Friction_Model/1(Friction_Torque) -> Sum6/1
  Sum6/1 -> Gain1/1
  Sum/1 -> Coulomb_Friction_Model1/1(Torque), Sum7/2
  Coulomb_Friction_Model1/1(Friction_Torque) -> Sum7/1
  Coulomb_Friction_Model1/2(reset velocity) -> Integrator2/2
  Integrator2/1 -> Sum8/2, Sum4/1, pod angular speed elevation/1
  Sum7/1 -> Gain2/1
  unballanced torque option1/1 -> Sum/3
  motor torque value pod/1 -> Coulomb_Friction_Model/4(motor torque value pod)
  torque load value pod/1 -> Coulomb_Friction_Model1/4(torque load value pod)
  external distribution/1 -> Sum9/1, Sum8/1
  Sum8/1 -> Coulomb_Friction_Model1/2(velocity), Sum1/2
  Integrator2/State -> Sum9/2
  Sum9/1 -> Coulomb_Friction_Model1/3(velocity state)

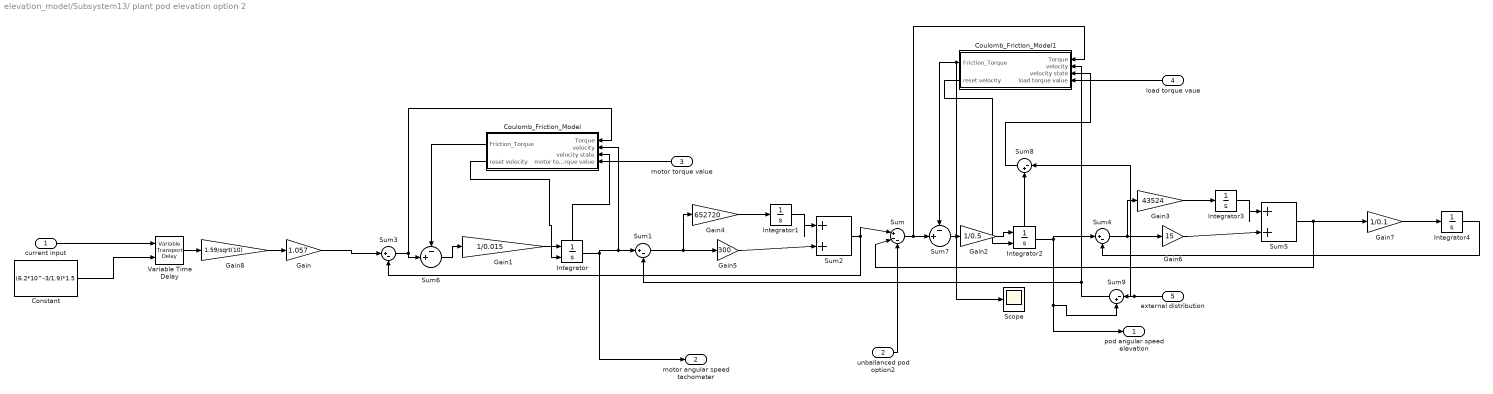
== system elevation_model/Subsystem13/ plant pod elevation option 2 ==
  current input : Inport
  unballanced pod option2 : Inport  Port=2
  motor torque value : Inport  Port=3
  load torque vaue : Inport  Port=4
  external distribution : Inport  Port=5
  Constant : Constant  Value=(6.2*10^-3/1.9)*1.5  SampleTime=-1
  Coulomb_Friction_Model : Subsystem
  Coulomb_Friction_Model1 : Subsystem
  Gain : Gain  Gain=1.057
  Gain1 : Gain  Gain=1/0.015
  Gain2 : Gain  Gain=1/0.5
  Gain3 : Gain  Gain=43524
  Gain4 : Gain  Gain=652720
  Gain5 : Gain  Gain=300
  Gain6 : Gain  Gain=15
  Gain7 : Gain  Gain=1/0.1
  Gain8 : Gain  Gain=1.59/sqrt(10)
  Integrator : Integrator  ExternalReset=rising  ShowStatePort=on  ZeroCross=off
  Integrator1 : Integrator
  Integrator2 : Integrator  ExternalReset=rising  ShowStatePort=on  ZeroCross=off
  Integrator3 : Integrator
  Integrator4 : Integrator
  Scope : Scope
  Sum : Sum  Inputs=|+--
  Sum1 : Sum  Inputs=|+-
  Sum2 : Sum  Inputs=|++
  Sum3 : Sum  Inputs=|+-
  Sum4 : Sum  Inputs=|+-
  Sum5 : Sum  Inputs=|++
  Sum6 : Sum  Inputs=-+|
  Sum7 : Sum  Inputs=-+|
  Sum8 : Sum  Inputs=|-+
  Sum9 : Sum  Inputs=|-+
  Variable Time Delay : VariableTransportDelay  MaximumDelay=10  TransDelayFeedthrough=on
  pod angular speed elevation : Outport
  "motor angular speed tachometer " : Outport  Port=2
  wires:
  Integrator3/1 -> Sum5/1
  Gain7/1 -> Integrator4/1
  Gain8/1 -> Gain/1
  Sum5/1 -> Gain7/1, Sum/2
  Gain6/1 -> Sum5/2
  Gain5/1 -> Sum2/2
  Integrator4/1 -> Sum4/2
  Gain/1 -> Sum3/1
  Sum1/1 -> Gain5/1, Gain4/1
  Sum4/1 -> Gain6/1, Gain3/1
  Integrator1/1 -> Sum2/1
  current input/1 -> Variable Time Delay/1
  Variable Time Delay/1 -> Gain8/1
  Constant/1 -> Variable Time Delay/2
  Sum2/1 -> Sum3/2, Sum/1
  Gain2/1 -> Integrator2/1
  Gain4/1 -> Integrator1/1
  Gain3/1 -> Integrator3/1
  Gain1/1 -> Integrator/1
  Integrator/1 -> Coulomb_Friction_Model/2(velocity), Sum1/1, "motor angular speed tachometer "/1
  Integrator/State -> Coulomb_Friction_Model/3(velocity state)
  Coulomb_Friction_Model/1(Friction_Torque) -> Sum6/1
  Sum3/1 -> Coulomb_Friction_Model/1(Torque), Sum6/2
  Coulomb_Friction_Model/2(reset velocity) -> Integrator/2
  Sum6/1 -> Gain1/1
  Coulomb_Friction_Model1/1(Friction_Torque) -> Sum7/1, Scope/1
  Sum/1 -> Sum7/2, Coulomb_Friction_Model1/1(Torque)
  Integrator2/1 -> Sum4/1, Sum9/2, pod angular speed elevation/1
  Coulomb_Friction_Model1/2(reset velocity) -> Integrator2/2
  Sum7/1 -> Gain2/1
  unballanced pod option2/1 -> Sum/3
  motor torque value/1 -> Coulomb_Friction_Model/4(motor torque value)
  load torque vaue/1 -> Coulomb_Friction_Model1/4(load torque value)
  Sum9/1 -> Coulomb_Friction_Model1/2(velocity), Sum1/2
  external distribution/1 -> Sum8/1, Sum9/1
  Integrator2/State -> Sum8/2
  Sum8/1 -> Coulomb_Friction_Model1/3(velocity state)

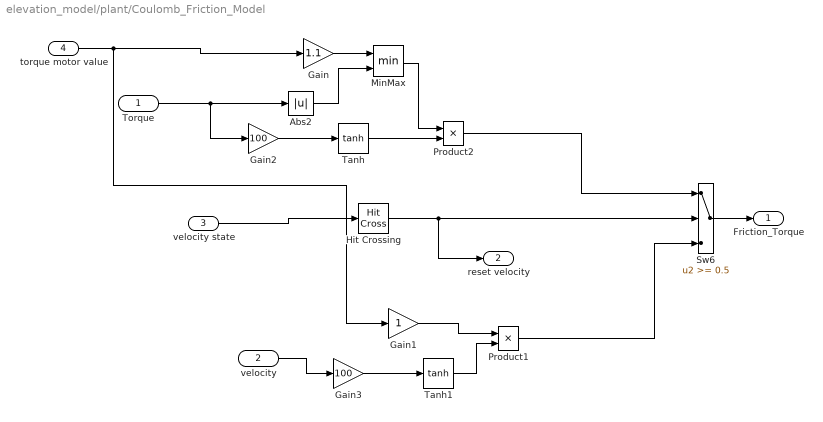
== system elevation_model/plant/Coulomb_Friction_Model ==
  Torque : Inport
  velocity : Inport  Port=2
  velocity state : Inport  Port=3
  torque motor value : Inport  Port=4
  Abs2 : Abs  ZeroCross=off
  Gain : Gain  Gain=1.1
  Gain1 : Gain
  Gain2 : Gain  Gain=100
  Gain3 : Gain  Gain=100
  Hit Crossing : HitCross  ZeroCross=off
  MinMax : MinMax  Inputs=2
  Product1 : Product  RndMeth=Zero
  Product2 : Product  RndMeth=Zero
  Sw6 : Switch  Threshold=0.5  ZeroCross=off  SaturateOnIntegerOverflow=on  InputSameDT=on
  Tanh : Trigonometry  Operator=tanh
  Tanh1 : Trigonometry  Operator=tanh
  Friction_Torque : Outport
  reset velocity : Outport  Port=2
  wires:
  Torque/1 -> Gain2/1, Abs2/1
  Sw6/1 -> Friction_Torque/1
  Hit Crossing/1 -> reset velocity/1, Sw6/2
  Abs2/1 -> MinMax/2
  MinMax/1 -> Product2/1
  Product2/1 -> Sw6/1
  Product1/1 -> Sw6/3
  velocity state/1 -> Hit Crossing/1
  Gain/1 -> MinMax/1
  Gain1/1 -> Product1/1
  Gain2/1 -> Tanh/1
  Tanh/1 -> Product2/2
  Gain3/1 -> Tanh1/1
  Tanh1/1 -> Product1/2
  velocity/1 -> Gain3/1
  torque motor value/1 -> Gain/1, Gain1/1

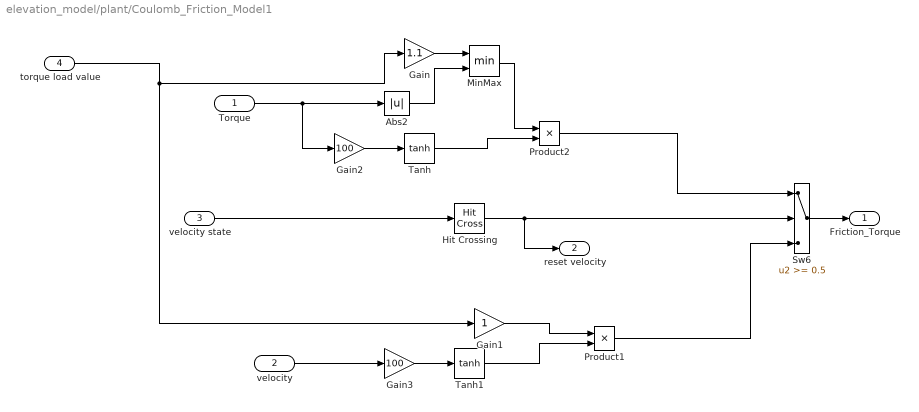
== system elevation_model/plant/Coulomb_Friction_Model1 ==
  Torque : Inport
  velocity : Inport  Port=2
  velocity state : Inport  Port=3
  torque load value : Inport  Port=4
  Abs2 : Abs  ZeroCross=off
  Gain : Gain  Gain=1.1
  Gain1 : Gain
  Gain2 : Gain  Gain=100
  Gain3 : Gain  Gain=100
  Hit Crossing : HitCross  ZeroCross=off
  MinMax : MinMax  Inputs=2
  Product1 : Product  RndMeth=Zero
  Product2 : Product  RndMeth=Zero
  Sw6 : Switch  Threshold=0.5  ZeroCross=off  SaturateOnIntegerOverflow=on  InputSameDT=on
  Tanh : Trigonometry  Operator=tanh
  Tanh1 : Trigonometry  Operator=tanh
  Friction_Torque : Outport
  reset velocity : Outport  Port=2
  wires:
  Torque/1 -> Gain2/1, Abs2/1
  Sw6/1 -> Friction_Torque/1
  Hit Crossing/1 -> reset velocity/1, Sw6/2
  Abs2/1 -> MinMax/2
  MinMax/1 -> Product2/1
  Product2/1 -> Sw6/1
  Product1/1 -> Sw6/3
  velocity state/1 -> Hit Crossing/1
  Gain/1 -> MinMax/1
  Gain1/1 -> Product1/1
  Gain2/1 -> Tanh/1
  Tanh/1 -> Product2/2
  Gain3/1 -> Tanh1/1
  velocity/1 -> Gain3/1
  Tanh1/1 -> Product1/2
  torque load value/1 -> Gain/1, Gain1/1

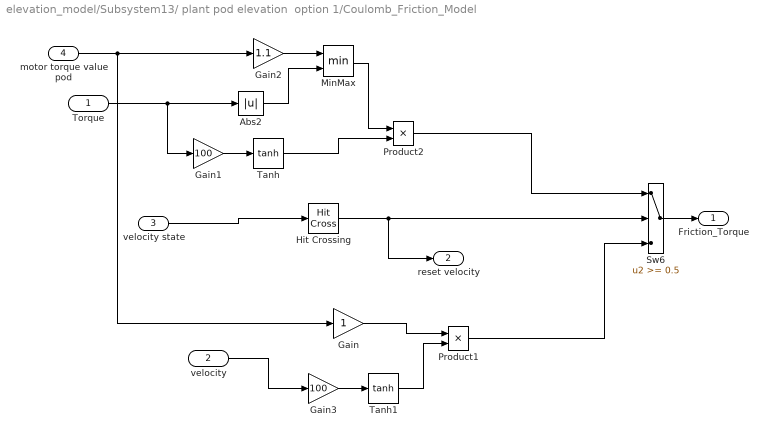
== system elevation_model/Subsystem13/ plant pod elevation  option 1/Coulomb_Friction_Model ==
  Torque : Inport
  velocity : Inport  Port=2
  velocity state : Inport  Port=3
  motor torque value pod : Inport  Port=4
  Abs2 : Abs  ZeroCross=off
  Gain : Gain
  Gain1 : Gain  Gain=100
  Gain2 : Gain  Gain=1.1
  Gain3 : Gain  Gain=100
  Hit Crossing : HitCross  ZeroCross=off
  MinMax : MinMax  Inputs=2
  Product1 : Product  RndMeth=Zero
  Product2 : Product  RndMeth=Zero
  Sw6 : Switch  Threshold=0.5  ZeroCross=off  SaturateOnIntegerOverflow=on  InputSameDT=on
  Tanh : Trigonometry  Operator=tanh
  Tanh1 : Trigonometry  Operator=tanh
  Friction_Torque : Outport
  reset velocity : Outport  Port=2
  wires:
  Torque/1 -> Gain1/1, Abs2/1
  Hit Crossing/1 -> reset velocity/1, Sw6/2
  Abs2/1 -> MinMax/2
  MinMax/1 -> Product2/1
  Product2/1 -> Sw6/1
  Product1/1 -> Sw6/3
  Gain2/1 -> MinMax/1
  velocity state/1 -> Hit Crossing/1
  Gain/1 -> Product1/1
  Gain1/1 -> Tanh/1
  Gain3/1 -> Tanh1/1
  Tanh/1 -> Product2/2
  Tanh1/1 -> Product1/2
  velocity/1 -> Gain3/1
  motor torque value pod/1 -> Gain2/1, Gain/1
  Sw6/1 -> Friction_Torque/1

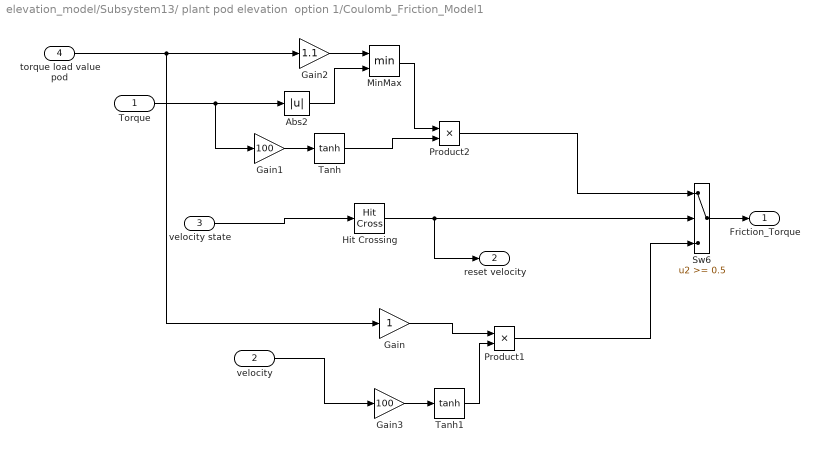
== system elevation_model/Subsystem13/ plant pod elevation  option 1/Coulomb_Friction_Model1 ==
  Torque : Inport
  velocity : Inport  Port=2
  velocity state : Inport  Port=3
  torque load value pod : Inport  Port=4
  Abs2 : Abs  ZeroCross=off
  Gain : Gain
  Gain1 : Gain  Gain=100
  Gain2 : Gain  Gain=1.1
  Gain3 : Gain  Gain=100
  Hit Crossing : HitCross  ZeroCross=off
  MinMax : MinMax  Inputs=2
  Product1 : Product  RndMeth=Zero
  Product2 : Product  RndMeth=Zero
  Sw6 : Switch  Threshold=0.5  ZeroCross=off  SaturateOnIntegerOverflow=on  InputSameDT=on
  Tanh : Trigonometry  Operator=tanh
  Tanh1 : Trigonometry  Operator=tanh
  Friction_Torque : Outport
  reset velocity : Outport  Port=2
  wires:
  Torque/1 -> Gain1/1, Abs2/1
  Sw6/1 -> Friction_Torque/1
  Hit Crossing/1 -> reset velocity/1, Sw6/2
  Abs2/1 -> MinMax/2
  MinMax/1 -> Product2/1
  Product2/1 -> Sw6/1
  Product1/1 -> Sw6/3
  Gain2/1 -> MinMax/1
  velocity state/1 -> Hit Crossing/1
  Gain/1 -> Product1/1
  Gain1/1 -> Tanh/1
  Tanh/1 -> Product2/2
  Gain3/1 -> Tanh1/1
  Tanh1/1 -> Product1/2
  velocity/1 -> Gain3/1
  torque load value pod/1 -> Gain/1, Gain2/1

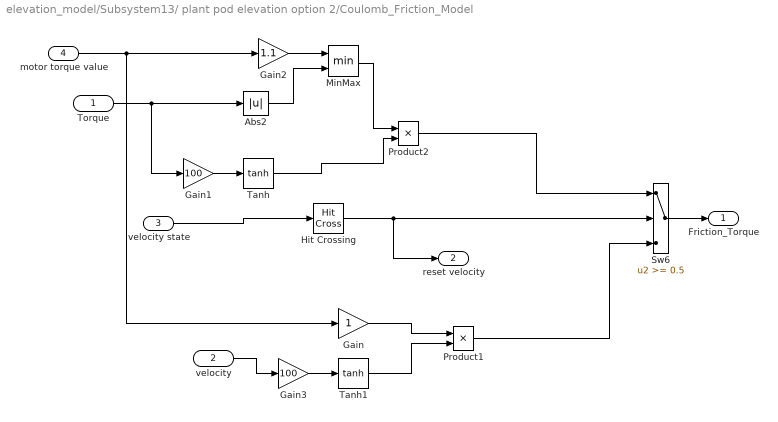
== system elevation_model/Subsystem13/ plant pod elevation option 2/Coulomb_Friction_Model ==
  Torque : Inport
  velocity : Inport  Port=2
  velocity state : Inport  Port=3
  motor torque value : Inport  Port=4
  Abs2 : Abs  ZeroCross=off
  Gain : Gain
  Gain1 : Gain  Gain=100
  Gain2 : Gain  Gain=1.1
  Gain3 : Gain  Gain=100
  Hit Crossing : HitCross  ZeroCross=off
  MinMax : MinMax  Inputs=2
  Product1 : Product  RndMeth=Zero
  Product2 : Product  RndMeth=Zero
  Sw6 : Switch  Threshold=0.5  ZeroCross=off  SaturateOnIntegerOverflow=on  InputSameDT=on
  Tanh : Trigonometry  Operator=tanh
  Tanh1 : Trigonometry  Operator=tanh
  Friction_Torque : Outport
  reset velocity : Outport  Port=2
  wires:
  Sw6/1 -> Friction_Torque/1
  Hit Crossing/1 -> reset velocity/1, Sw6/2
  Abs2/1 -> MinMax/2
  MinMax/1 -> Product2/1
  Product2/1 -> Sw6/1
  Product1/1 -> Sw6/3
  Gain2/1 -> MinMax/1
  velocity state/1 -> Hit Crossing/1
  Gain/1 -> Product1/1
  Gain1/1 -> Tanh/1
  Tanh/1 -> Product2/2
  Torque/1 -> Gain1/1, Abs2/1
  Gain3/1 -> Tanh1/1
  Tanh1/1 -> Product1/2
  velocity/1 -> Gain3/1
  motor torque value/1 -> Gain2/1, Gain/1

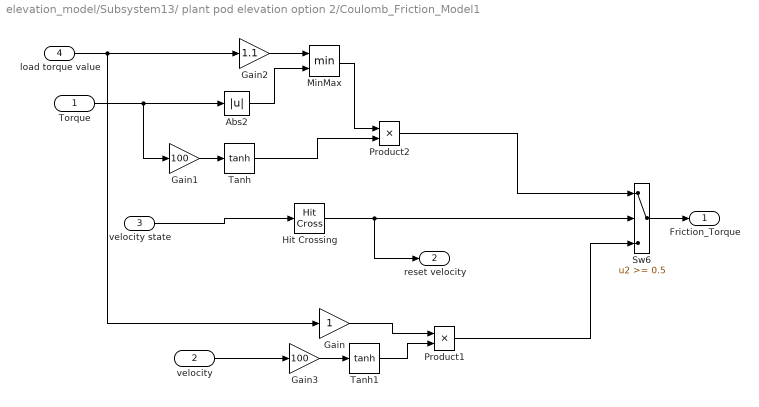
== system elevation_model/Subsystem13/ plant pod elevation option 2/Coulomb_Friction_Model1 ==
  Torque : Inport
  velocity : Inport  Port=2
  velocity state : Inport  Port=3
  load torque value : Inport  Port=4
  Abs2 : Abs  ZeroCross=off
  Gain : Gain
  Gain1 : Gain  Gain=100
  Gain2 : Gain  Gain=1.1
  Gain3 : Gain  Gain=100
  Hit Crossing : HitCross  ZeroCross=off
  MinMax : MinMax  Inputs=2
  Product1 : Product  RndMeth=Zero
  Product2 : Product  RndMeth=Zero
  Sw6 : Switch  Threshold=0.5  ZeroCross=off  SaturateOnIntegerOverflow=on  InputSameDT=on
  Tanh : Trigonometry  Operator=tanh
  Tanh1 : Trigonometry  Operator=tanh
  Friction_Torque : Outport
  reset velocity : Outport  Port=2
  wires:
  Torque/1 -> Gain1/1, Abs2/1
  Sw6/1 -> Friction_Torque/1
  Hit Crossing/1 -> reset velocity/1, Sw6/2
  Abs2/1 -> MinMax/2
  MinMax/1 -> Product2/1
  Product2/1 -> Sw6/1
  Product1/1 -> Sw6/3
  Gain2/1 -> MinMax/1
  velocity state/1 -> Hit Crossing/1
  Gain/1 -> Product1/1
  Gain1/1 -> Tanh/1
  Tanh/1 -> Product2/2
  Gain3/1 -> Tanh1/1
  velocity/1 -> Gain3/1
  Tanh1/1 -> Product1/2
  load torque value/1 -> Gain2/1, Gain/1
